simulink model "AM"  (R2020b)
settings: Solver=VariableStepAuto  StartTime=0.0  StopTime=10.0  RelTol=1e-3
libraries: dspvision x3, audiosources x2, dspfdesign x2
settings Model: Creator=MinsooKang  LastModifiedBy=MinsooKang

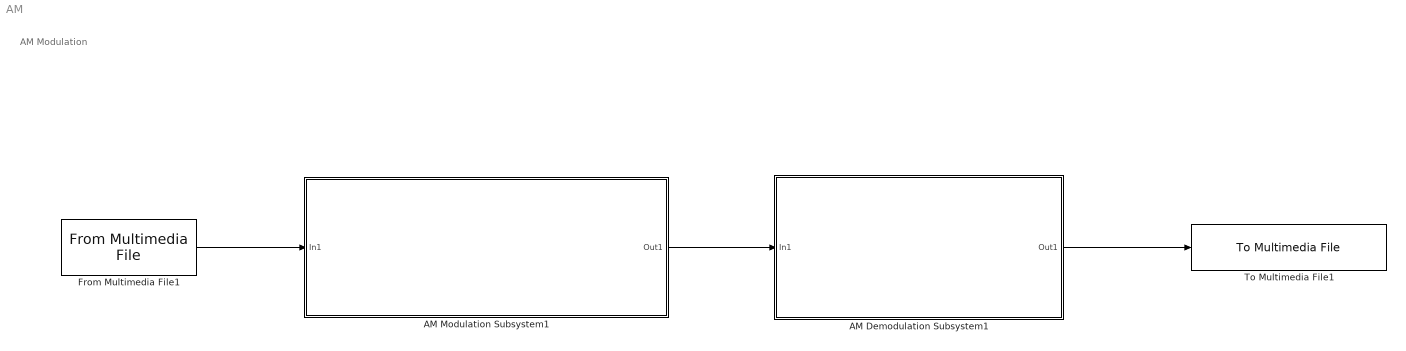
== system AM ==
  note: AM Modulation
  " AM Demodulation Subsystem1" : Subsystem
  AM Modulation Subsystem1 : Subsystem
  From Multimedia File1 : dspvision/From Multimedia File  inputFilename=C:\Users\MinsooKang\Desktop\matlab\audio.flac  readRange=[1 Inf]  loop=on  numPlays=inf  outputStreams=Audio only  videoDataType=single  audioDataType=double  inheritSampleTime=on  userDefinedSampleTime=1/30  noAudioOutput=off  isIntensityVideo=off  fourcc=RGB  colorVideoFormat=Separate color signals  outputEOF=off  dataOrg=Column-major  audioFrameSize=1024  computeAudioFrameSize=off  outSamplingMode=Sample based
  To Multimedia File1 : dspvision/To Multimedia File  outputFilename=AM_demodulated.wav  streamSelection=Audio only  videoCompressor=None (uncompressed)  audioCompressor=None (uncompressed)  imagePorts=Separate color signals  fileType=WAV  audioDatatype=32-bit float  fourcc=RGB  videoQuality=75  mj2000CompFactor=10
  wires:
  AM Modulation Subsystem1/1(Out1) -> " AM Demodulation Subsystem1"/1(In1)
  From Multimedia File1/1 -> AM Modulation Subsystem1/1(In1)
  " AM Demodulation Subsystem1"/1(Out1) -> To Multimedia File1/1

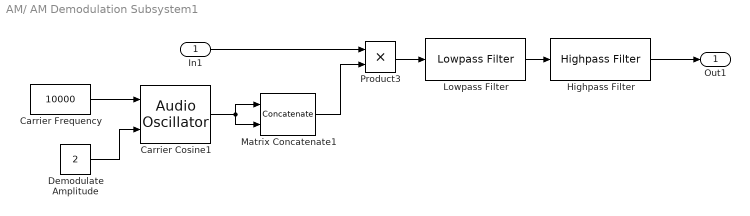
== system AM/ AM Demodulation Subsystem1 ==
  In1 : Inport
  Carrier Cosine1 : audiosources/Audio Oscillator  FrequencyPort=on  Frequency=100  AmplitudePort=on  Amplitude=1  DCOffsetPort=off  PhaseOffset=0.25  DCOffset=0  WidthPort=off  Width=1  DutyCyclePort=off  DutyCycle=0.5  SampsPerFrame=1024  Fs=44100  OutputDataType=double  SimulateUsing=Code generation
      settings: SourceProductBaseCode=AU  SignalType=sine
  Carrier Frequency : Constant  Value=10000
  Demodulate Amplitude : Constant  Value=2
  Highpass Filter : dspfdesign/Highpass Filter  FilterType=FIR  DesignForMinimumOrder=on  FilterOrder=50  StopbandFrequency=20  PassbandFrequency=50  StopbandAttenuation=80  PassbandRipple=0.1  InheritSampleRate=off  SampleRate=44100  SimulateUsing=Interpreted execution  roundingMode=Floor  coeffsDataTypeStr=fixdt(1,16)
  Lowpass Filter : dspfdesign/Lowpass Filter  FilterType=FIR  DesignForMinimumOrder=on  FilterOrder=50  PassbandFrequency=1500  StopbandFrequency=1600  PassbandRipple=0.1  StopbandAttenuation=80  InheritSampleRate=off  SampleRate=44100  SimulateUsing=Interpreted execution  roundingMode=Floor  coeffsDataTypeStr=fixdt(1,16)
  Matrix Concatenate1 : Concatenate  Mode=Multidimensional array  ConcatenateDimension=2
  Product3 : Product
  Out1 : Outport
  wires:
  Highpass Filter/1 -> Out1/1
  Lowpass Filter/1 -> Highpass Filter/1
  Matrix Concatenate1/1 -> Product3/2
  Product3/1 -> Lowpass Filter/1
  Carrier Cosine1/1 -> Matrix Concatenate1/2, Matrix Concatenate1/1
  In1/1 -> Product3/1
  Carrier Frequency/1 -> Carrier Cosine1/1
  Demodulate Amplitude/1 -> Carrier Cosine1/2

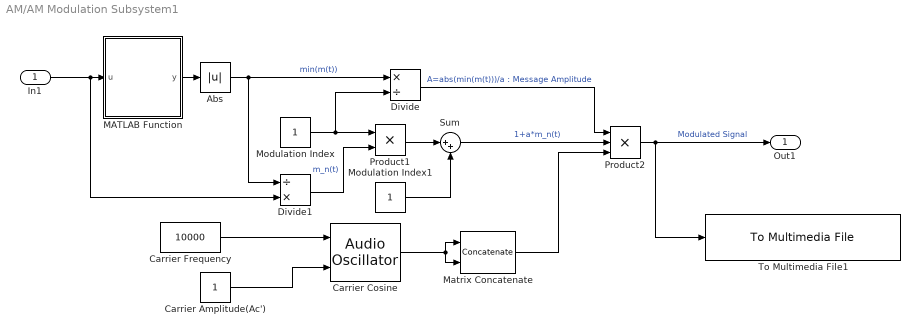
== system AM/AM Modulation Subsystem1 ==
  In1 : Inport
  Abs : Abs
  Carrier Amplitude(Ac') : Constant
  Carrier Cosine : audiosources/Audio Oscillator  FrequencyPort=on  Frequency=100  AmplitudePort=on  Amplitude=1  DCOffsetPort=off  PhaseOffset=0.25  DCOffset=0  WidthPort=off  Width=1  DutyCyclePort=off  DutyCycle=0.5  SampsPerFrame=1024  Fs=44100  OutputDataType=double  SimulateUsing=Code generation
      settings: SourceProductBaseCode=AU  SignalType=sine
  Carrier Frequency : Constant  Value=10000
  Divide : Product  Inputs=*/
  Divide1 : Product  Inputs=/*
  MATLAB Function : MATLAB Function  TreatAsAtomicUnit=on
  Matrix Concatenate : Concatenate  Mode=Multidimensional array  ConcatenateDimension=2
  Modulation Index : Constant
  Modulation Index1 : Constant
  Product1 : Product
  Product2 : Product  Inputs=3
  Sum : Sum  Inputs=|++
  To Multimedia File1 : dspvision/To Multimedia File  outputFilename=C:\Users\MinsooKang\Desktop\matlab\AM_modulated.wav  streamSelection=Audio only  videoCompressor=None (uncompressed)  audioCompressor=None (uncompressed)  imagePorts=Separate color signals  fileType=WAV  audioDatatype=32-bit float  fourcc=RGB  videoQuality=75  mj2000CompFactor=10
  Out1 : Outport
  wires:
  Carrier Frequency/1 -> Carrier Cosine/1
  Carrier Amplitude(Ac')/1 -> Carrier Cosine/2
  Product2/1 -> To Multimedia File1/1, Out1/1  "Modulated Signal"
  Abs/1 -> Divide1/1, Divide/1  "min(m(t))"
  In1/1 -> Divide1/2, MATLAB Function/1(u)
  Carrier Cosine/1 -> Matrix Concatenate/2, Matrix Concatenate/1
  Modulation Index/1 -> Divide/2, Product1/1
  Divide1/1 -> Product1/2  "m_n(t)"
  Matrix Concatenate/1 -> Product2/3
  Sum/1 -> Product2/2  "1+a*m_n(t)"
  Divide/1 -> Product2/1  "A=abs(min(m(t)))/a : Message Amplitude"
  Product1/1 -> Sum/1
  MATLAB Function/1(y) -> Abs/1
  Modulation Index1/1 -> Sum/2

== matlab function AM/AM Modulation Subsystem1/MATLAB Function ==
  data: u input; y output
function y = min_columns(u)
min_val=min(u);
[rows,cols]=size(u);
y= repmat(min_val,rows,1);
end
